simulink model "RichaLaika"  (R2025b)
settings: Solver=VariableStepAuto  StartTime=0.0  StopTime=10.0  RelTol=1e-3
undefined symbols (not defined in the file): ActivationSignal, ChargingWire, DataIN, DataOUT, OutputWire, SwitchSignal, TriggerSignal
settings Model: Creator=jakeo  LastModifiedBy=Richa

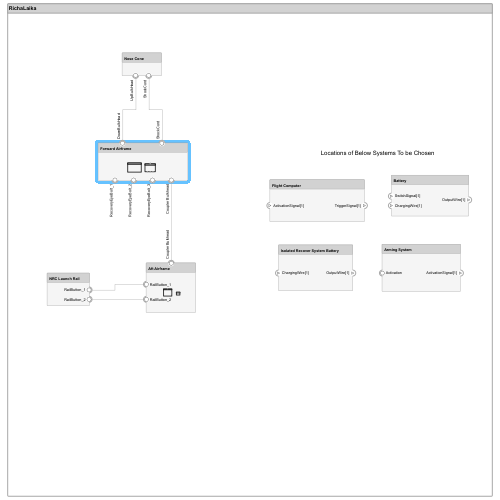
[thumbnail: Simulink's stored preview of the top-level diagram]
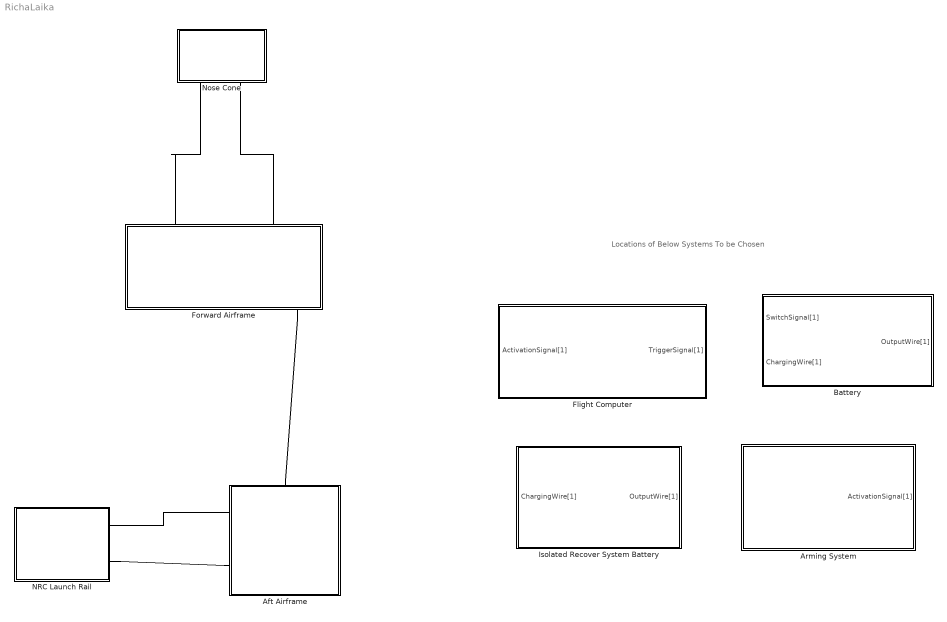
== system RichaLaika ==
  note: Locations of Below Systems To be Chosen
  Aft Airframe : Subsystem
      settings: PortSchema="{\"entries\":[{\"content\":{\"headerSize\":26,\"margin\":15,\"minimumSpacing\":25,\"sides\":[{\"content\":{\"connectorIds\":[\"LConn1\",\"LConn2\"]},\"type\":\"ConnectorPlacement.EquallySpacedRectSide\",\"uuid\":\"03e957df-4bae-46ab-9d0d-48f80a496ac5\"},{\"content\":{\"side\":\"RIGHT\"},\"type\":\"ConnectorPlacement.EquallySpacedRectSide\",\"uuid\":\"d2433d43-ba0e-4345-8a8e-99b57dcef125\"},{\"content\":{\"connectorIds\":[\"LConn3\"],\"side\":\"TOP\"},\"type\":\"ConnectorPlacement.EquallySpacedRectSide\",\"uuid\":\"84844adf-0e3d-439c-a28c-7cf27e8d243a\"},{\"content\":{\"side\":\"BOTTOM\"},\"type\":\"ConnectorPlacement.EquallySpacedRectSide\",\"uuid\":\"3d019cf0-7990-47c2-88c6-9af96c612354\"}]},\"type\":\"ConnectorPlacement.EquallySpacedConnector\",\"uuid\":\"9b26577b-50b2-4983-8f3c-4df87f23ba49\"}],\"packageUris\":[\"http://schema.mathworks.com/mf0/Connector/R2020b\"],\"version\":\"1.0\"}"
  Arming System : Subsystem
      settings: PortSchema="{\"entries\":[{\"content\":{\"headerSize\":26,\"margin\":15,\"minimumSpacing\":25,\"sides\":[{\"content\":{\"connectorIds\":[\"LConn1\"]},\"type\":\"ConnectorPlacement.EquallySpacedRectSide\",\"uuid\":\"6f4db608-f49c-4d1a-85cc-b66ec62c2f96\"},{\"content\":{\"connectorIds\":[\"Out1\"],\"side\":\"RIGHT\"},\"type\":\"ConnectorPlacement.EquallySpacedRectSide\",\"uuid\":\"3e275c67-1c5c-46cd-973f-75adcfca9e5d\"},{\"content\":{\"side\":\"TOP\"},\"type\":\"ConnectorPlacement.EquallySpacedRectSide\",\"uuid\":\"88fdcd36-c2bf-423f-a1bd-8e2b1c2ac438\"}]},\"type\":\"ConnectorPlacement.EquallySpacedConnector\",\"uuid\":\"596a3d77-8add-49e5-be48-e23e6a2b115a\"}],\"packageUris\":[\"http://schema.mathworks.com/mf0/Connector/R2020b\"],\"version\":\"1.0\"}"
  Battery : Subsystem
      settings: PortSchema="{\"entries\":[{\"content\":{\"headerSize\":26,\"margin\":15,\"minimumSpacing\":25,\"sides\":[{\"content\":{\"connectorIds\":[\"In1\",\"In2\"]},\"type\":\"ConnectorPlacement.EquallySpacedRectSide\",\"uuid\":\"03e957df-4bae-46ab-9d0d-48f80a496ac5\"},{\"content\":{\"connectorIds\":[\"Out1\"],\"side\":\"RIGHT\"},\"type\":\"ConnectorPlacement.EquallySpacedRectSide\",\"uuid\":\"d2433d43-ba0e-4345-8a8e-99b57dcef125\"},{\"content\":{\"side\":\"TOP\"},\"type\":\"ConnectorPlacement.EquallySpacedRectSide\",\"uuid\":\"84844adf-0e3d-439c-a28c-7cf27e8d243a\"}]},\"type\":\"ConnectorPlacement.EquallySpacedConnector\",\"uuid\":\"9b26577b-50b2-4983-8f3c-4df87f23ba49\"}],\"packageUris\":[\"http://schema.mathworks.com/mf0/Connector/R2020b\"],\"version\":\"1.0\"}"
  Flight Computer : Subsystem
      settings: PortSchema="{\"entries\":[{\"content\":{\"headerSize\":26,\"margin\":15,\"minimumSpacing\":25,\"sides\":[{\"content\":{\"connectorIds\":[\"In1\"]},\"type\":\"ConnectorPlacement.EquallySpacedRectSide\",\"uuid\":\"6f4db608-f49c-4d1a-85cc-b66ec62c2f96\"},{\"content\":{\"connectorIds\":[\"Out1\"],\"side\":\"RIGHT\"},\"type\":\"ConnectorPlacement.EquallySpacedRectSide\",\"uuid\":\"3e275c67-1c5c-46cd-973f-75adcfca9e5d\"},{\"content\":{\"side\":\"TOP\"},\"type\":\"ConnectorPlacement.EquallySpacedRectSide\",\"uuid\":\"88fdcd36-c2bf-423f-a1bd-8e2b1c2ac438\"}]},\"type\":\"ConnectorPlacement.EquallySpacedConnector\",\"uuid\":\"596a3d77-8add-49e5-be48-e23e6a2b115a\"}],\"packageUris\":[\"http://schema.mathworks.com/mf0/Connector/R2020b\"],\"version\":\"1.0\"}"
  Forward Airframe : Subsystem
      settings: PortSchema="{\"entries\":[{\"content\":{\"headerSize\":26,\"margin\":15,\"minimumSpacing\":25,\"sides\":[{\"content\":{},\"type\":\"ConnectorPlacement.EquallySpacedRectSide\",\"uuid\":\"03e957df-4bae-46ab-9d0d-48f80a496ac5\"},{\"content\":{\"side\":\"RIGHT\"},\"type\":\"ConnectorPlacement.EquallySpacedRectSide\",\"uuid\":\"d2433d43-ba0e-4345-8a8e-99b57dcef125\"},{\"content\":{\"connectorIds\":[\"LConn2\",\"LConn1\"],\"side\":\"TOP\"},\"type\":\"ConnectorPlacement.EquallySpacedRectSide\",\"uuid\":\"84844adf-0e3d-439c-a28c-7cf27e8d243a\"},{\"content\":{\"connectorIds\":[\"RConn2\",\"RConn3\",\"RConn4\",\"RConn1\"],\"side\":\"BOTTOM\"},\"type\":\"ConnectorPlacement.EquallySpacedRectSide\",\"uuid\":\"7d79bddd-aaf5-48a9-85da-385393746c36\"}]},\"type\":\"ConnectorPlacement.EquallySpacedConnector\",\"uuid\":\"9b26577b-50b2-4983-8f3c-4df87f23ba49\"}],\"packageUris\":[\"http://schema.mathworks.com/mf0/Connector/R2020b\"],\"version\":\"1.0\"}"
  Isolated Recover System Battery : Subsystem
      settings: PortSchema="{\"entries\":[{\"content\":{\"headerSize\":26,\"margin\":15,\"minimumSpacing\":25,\"sides\":[{\"content\":{\"connectorIds\":[\"In1\"]},\"type\":\"ConnectorPlacement.EquallySpacedRectSide\",\"uuid\":\"6f4db608-f49c-4d1a-85cc-b66ec62c2f96\"},{\"content\":{\"connectorIds\":[\"Out1\"],\"side\":\"RIGHT\"},\"type\":\"ConnectorPlacement.EquallySpacedRectSide\",\"uuid\":\"3e275c67-1c5c-46cd-973f-75adcfca9e5d\"},{\"content\":{\"side\":\"TOP\"},\"type\":\"ConnectorPlacement.EquallySpacedRectSide\",\"uuid\":\"88fdcd36-c2bf-423f-a1bd-8e2b1c2ac438\"}]},\"type\":\"ConnectorPlacement.EquallySpacedConnector\",\"uuid\":\"596a3d77-8add-49e5-be48-e23e6a2b115a\"}],\"packageUris\":[\"http://schema.mathworks.com/mf0/Connector/R2020b\"],\"version\":\"1.0\"}"
  NRC Launch Rail : Subsystem
      settings: PortSchema="{\"entries\":[{\"content\":{\"headerSize\":26,\"margin\":15,\"minimumSpacing\":25,\"sides\":[{\"content\":{},\"type\":\"ConnectorPlacement.EquallySpacedRectSide\",\"uuid\":\"6f4db608-f49c-4d1a-85cc-b66ec62c2f96\"},{\"content\":{\"connectorIds\":[\"RConn1\",\"RConn2\"],\"side\":\"RIGHT\"},\"type\":\"ConnectorPlacement.EquallySpacedRectSide\",\"uuid\":\"3e275c67-1c5c-46cd-973f-75adcfca9e5d\"},{\"content\":{\"side\":\"TOP\"},\"type\":\"ConnectorPlacement.EquallySpacedRectSide\",\"uuid\":\"88fdcd36-c2bf-423f-a1bd-8e2b1c2ac438\"}]},\"type\":\"ConnectorPlacement.EquallySpacedConnector\",\"uuid\":\"596a3d77-8add-49e5-be48-e23e6a2b115a\"}],\"packageUris\":[\"http://schema.mathworks.com/mf0/Connector/R2020b\"],\"version\":\"1.0\"}"
  Nose Cone : Subsystem
      settings: PortSchema="{\"entries\":[{\"content\":{\"headerSize\":26,\"margin\":15,\"minimumSpacing\":25,\"sides\":[{\"content\":{},\"type\":\"ConnectorPlacement.EquallySpacedRectSide\",\"uuid\":\"03e957df-4bae-46ab-9d0d-48f80a496ac5\"},{\"content\":{\"side\":\"RIGHT\"},\"type\":\"ConnectorPlacement.EquallySpacedRectSide\",\"uuid\":\"d2433d43-ba0e-4345-8a8e-99b57dcef125\"},{\"content\":{\"side\":\"TOP\"},\"type\":\"ConnectorPlacement.EquallySpacedRectSide\",\"uuid\":\"84844adf-0e3d-439c-a28c-7cf27e8d243a\"},{\"content\":{\"connectorIds\":[\"RConn1\",\"LConn1\"],\"side\":\"BOTTOM\"},\"type\":\"ConnectorPlacement.EquallySpacedRectSide\",\"uuid\":\"52e1799e-3f90-4e46-b959-6af2ed3cd00a\"}]},\"type\":\"ConnectorPlacement.EquallySpacedConnector\",\"uuid\":\"9b26577b-50b2-4983-8f3c-4df87f23ba49\"}],\"packageUris\":[\"http://schema.mathworks.com/mf0/Connector/R2020b\"],\"version\":\"1.0\"}"
  connections:
  Nose Cone/LConn1 -- Forward Airframe/LConn1
  Nose Cone/RConn1 -- Forward Airframe/LConn2
  NRC Launch Rail/RConn1 -- Aft Airframe/LConn1
  NRC Launch Rail/RConn2 -- Aft Airframe/LConn2
  Forward Airframe/RConn1 -- Aft Airframe/LConn3

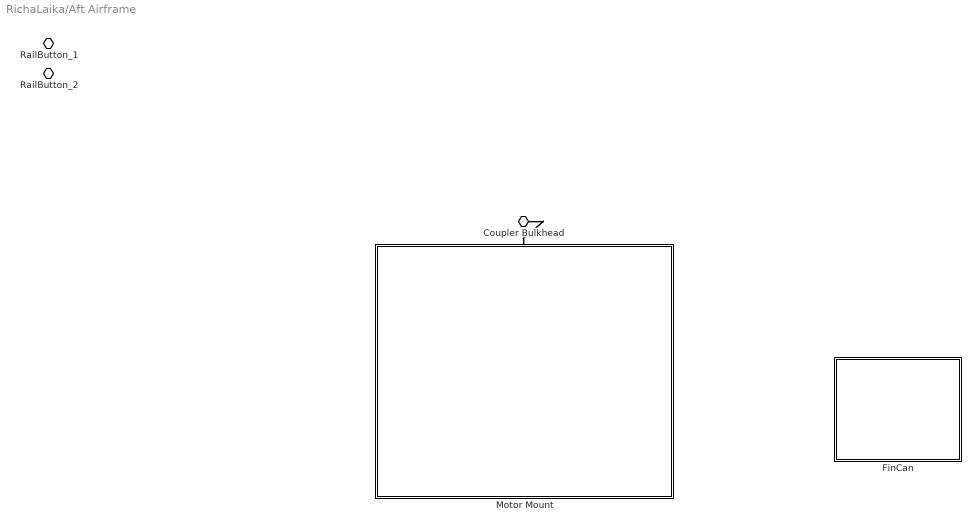
== system RichaLaika/Aft Airframe ==
  FinCan : Subsystem
      settings: PortSchema="{\"entries\":[{\"content\":{\"headerSize\":26,\"margin\":15,\"minimumSpacing\":25,\"sides\":[{\"content\":{},\"type\":\"ConnectorPlacement.EquallySpacedRectSide\",\"uuid\":\"b8130898-a228-4777-928b-c45fd71fae12\"},{\"content\":{\"side\":\"RIGHT\"},\"type\":\"ConnectorPlacement.EquallySpacedRectSide\",\"uuid\":\"2e534d82-eb77-4958-a6c7-3df50b0f76b8\"},{\"content\":{\"connectorIds\":[\"LConn1\",\"LConn2\",\"LConn3\",\"LConn4\"],\"side\":\"TOP\"},\"type\":\"ConnectorPlacement.EquallySpacedRectSide\",\"uuid\":\"3377e7dd-a415-4e95-88ef-4d0f5ef1cb04\"}]},\"type\":\"ConnectorPlacement.EquallySpacedConnector\",\"uuid\":\"f74309f9-da3e-4b22-b86a-0a2c471e6b03\"}],\"packageUris\":[\"http://schema.mathworks.com/mf0/Connector/R2020b\"],\"version\":\"1.0\"}"
  Motor Mount : Subsystem
      settings: PortSchema="{\"entries\":[{\"content\":{\"headerSize\":26,\"margin\":15,\"minimumSpacing\":25,\"sides\":[{\"content\":{},\"type\":\"ConnectorPlacement.EquallySpacedRectSide\",\"uuid\":\"31a1afce-5e8d-4ecd-8541-15d1c40c1f45\"},{\"content\":{\"connectorIds\":[\"LConn2\"],\"side\":\"RIGHT\"},\"type\":\"ConnectorPlacement.EquallySpacedRectSide\",\"uuid\":\"3ed7ed21-4334-432f-9367-bfee11c65601\"},{\"content\":{\"connectorIds\":[\"LConn1\"],\"side\":\"TOP\"},\"type\":\"ConnectorPlacement.EquallySpacedRectSide\",\"uuid\":\"099656eb-739b-474e-8ddd-dbd0ceba9a2b\"}]},\"type\":\"ConnectorPlacement.EquallySpacedConnector\",\"uuid\":\"a8320310-5044-4b61-8848-b99dff184188\"}],\"packageUris\":[\"http://schema.mathworks.com/mf0/Connector/R2020b\"],\"version\":\"1.0\"}"
  RailButton_1 : PMIOPort  Side=Left
  RailButton_2 : PMIOPort  Port=2  Side=Left
  Coupler Bulkhead : PMIOPort  Port=3  Side=Left
  connections:
  Coupler Bulkhead/RConn1 -- Motor Mount/LConn1

== system RichaLaika/Arming System ==
  Activation : PMIOPort  Side=Left
  Bus Element Out1 : Outport  PortName=ActivationSignal[1]

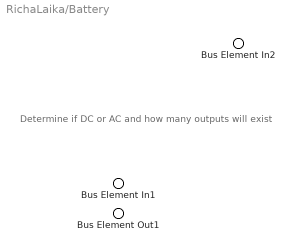
== system RichaLaika/Battery ==
  note: Determine if DC or AC and how many outputs will exist
  Bus Element In2 : Inport  PortName=SwitchSignal[1]
  Bus Element In1 : Inport  Port=2  PortName=ChargingWire[1]
  Bus Element Out1 : Outport  PortName=OutputWire[1]

== system RichaLaika/Flight Computer ==
  Bus Element In1 : Inport  PortName=ActivationSignal[1]
  Bus Element Out1 : Outport  PortName=TriggerSignal[1]

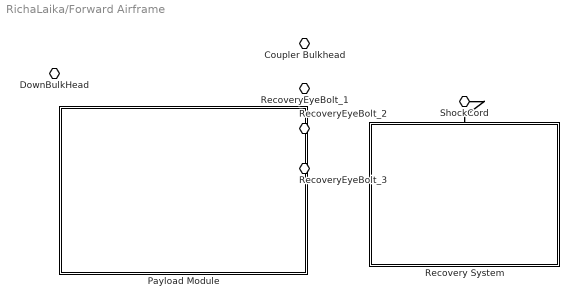
== system RichaLaika/Forward Airframe ==
  Payload Module : Subsystem
      settings: PortSchema="{\"entries\":[{\"content\":{\"headerSize\":26,\"margin\":15,\"minimumSpacing\":25,\"sides\":[{\"content\":{},\"type\":\"ConnectorPlacement.EquallySpacedRectSide\",\"uuid\":\"31a1afce-5e8d-4ecd-8541-15d1c40c1f45\"},{\"content\":{\"side\":\"RIGHT\"},\"type\":\"ConnectorPlacement.EquallySpacedRectSide\",\"uuid\":\"3ed7ed21-4334-432f-9367-bfee11c65601\"},{\"content\":{\"side\":\"TOP\"},\"type\":\"ConnectorPlacement.EquallySpacedRectSide\",\"uuid\":\"099656eb-739b-474e-8ddd-dbd0ceba9a2b\"}]},\"type\":\"ConnectorPlacement.EquallySpacedConnector\",\"uuid\":\"a8320310-5044-4b61-8848-b99dff184188\"}],\"packageUris\":[\"http://schema.mathworks.com/mf0/Connector/R2020b\"],\"version\":\"1.0\"}"
  Recovery System : Subsystem
      settings: PortSchema="{\"entries\":[{\"content\":{\"headerSize\":26,\"margin\":15,\"minimumSpacing\":25,\"sides\":[{\"content\":{},\"type\":\"ConnectorPlacement.EquallySpacedRectSide\",\"uuid\":\"31a1afce-5e8d-4ecd-8541-15d1c40c1f45\"},{\"content\":{\"side\":\"RIGHT\"},\"type\":\"ConnectorPlacement.EquallySpacedRectSide\",\"uuid\":\"3ed7ed21-4334-432f-9367-bfee11c65601\"},{\"content\":{\"connectorIds\":[\"LConn1\"],\"side\":\"TOP\"},\"type\":\"ConnectorPlacement.EquallySpacedRectSide\",\"uuid\":\"099656eb-739b-474e-8ddd-dbd0ceba9a2b\"},{\"content\":{\"connectorIds\":[\"RConn3\",\"RConn1\",\"RConn2\"],\"side\":\"BOTTOM\"},\"type\":\"ConnectorPlacement.EquallySpacedRectSide\",\"uuid\":\"aa9f3616-ef86-4a01-82fa-8dfdf1ff0ef2\"}]},\"type\":\"ConnectorPlacement.EquallySpacedConnector\",\"uuid\":\"a8320310-5044-4b61-8848-b99dff184188\"}],\"packageUris\":[\"http://schema.mathworks.com/mf0/Connector/R2020b\"],\"version\":\"1.0\"}"
  ShockCord : PMIOPort  Side=Left
  DownBulkHead : PMIOPort  Port=2  Side=Left
  Coupler Bulkhead : PMIOPort  Port=3  Side=Right
  RecoveryEyeBolt_1 : PMIOPort  Port=4  Side=Right
  RecoveryEyeBolt_2 : PMIOPort  Port=5  Side=Right
  RecoveryEyeBolt_3 : PMIOPort  Port=6  Side=Right
  connections:
  ShockCord/RConn1 -- Recovery System/LConn1

== system RichaLaika/Isolated Recover System Battery ==
  Bus Element In1 : Inport  PortName=ChargingWire[1]
  Bus Element Out1 : Outport  PortName=OutputWire[1]

== system RichaLaika/NRC Launch Rail ==
  RailButton_1 : PMIOPort  Side=Right
  RailButton_2 : PMIOPort  Port=2  Side=Right

== system RichaLaika/Nose Cone ==
  ShockCord : PMIOPort  Side=Left
  UpBulkHead : PMIOPort  Port=2  Side=Right

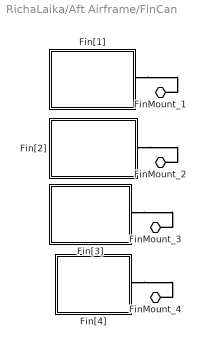
== system RichaLaika/Aft Airframe/FinCan ==
  Fin[1] : Subsystem
      settings: PortSchema="{\"entries\":[{\"content\":{\"headerSize\":26,\"margin\":15,\"minimumSpacing\":25,\"sides\":[{\"content\":{},\"type\":\"ConnectorPlacement.EquallySpacedRectSide\",\"uuid\":\"03e957df-4bae-46ab-9d0d-48f80a496ac5\"},{\"content\":{\"connectorIds\":[\"LConn1\"],\"side\":\"RIGHT\"},\"type\":\"ConnectorPlacement.EquallySpacedRectSide\",\"uuid\":\"d2433d43-ba0e-4345-8a8e-99b57dcef125\"},{\"content\":{\"side\":\"TOP\"},\"type\":\"ConnectorPlacement.EquallySpacedRectSide\",\"uuid\":\"84844adf-0e3d-439c-a28c-7cf27e8d243a\"}]},\"type\":\"ConnectorPlacement.EquallySpacedConnector\",\"uuid\":\"9b26577b-50b2-4983-8f3c-4df87f23ba49\"}],\"packageUris\":[\"http://schema.mathworks.com/mf0/Connector/R2020b\"],\"version\":\"1.0\"}"
  Fin[2] : Subsystem
      settings: PortSchema="{\"entries\":[{\"content\":{\"headerSize\":26,\"margin\":15,\"minimumSpacing\":25,\"sides\":[{\"content\":{},\"type\":\"ConnectorPlacement.EquallySpacedRectSide\",\"uuid\":\"03e957df-4bae-46ab-9d0d-48f80a496ac5\"},{\"content\":{\"connectorIds\":[\"LConn1\"],\"side\":\"RIGHT\"},\"type\":\"ConnectorPlacement.EquallySpacedRectSide\",\"uuid\":\"d2433d43-ba0e-4345-8a8e-99b57dcef125\"},{\"content\":{\"side\":\"TOP\"},\"type\":\"ConnectorPlacement.EquallySpacedRectSide\",\"uuid\":\"84844adf-0e3d-439c-a28c-7cf27e8d243a\"}]},\"type\":\"ConnectorPlacement.EquallySpacedConnector\",\"uuid\":\"9b26577b-50b2-4983-8f3c-4df87f23ba49\"}],\"packageUris\":[\"http://schema.mathworks.com/mf0/Connector/R2020b\"],\"version\":\"1.0\"}"
  Fin[3] : Subsystem
      settings: PortSchema="{\"entries\":[{\"content\":{\"headerSize\":26,\"margin\":15,\"minimumSpacing\":25,\"sides\":[{\"content\":{},\"type\":\"ConnectorPlacement.EquallySpacedRectSide\",\"uuid\":\"03e957df-4bae-46ab-9d0d-48f80a496ac5\"},{\"content\":{\"connectorIds\":[\"LConn1\"],\"side\":\"RIGHT\"},\"type\":\"ConnectorPlacement.EquallySpacedRectSide\",\"uuid\":\"d2433d43-ba0e-4345-8a8e-99b57dcef125\"},{\"content\":{\"side\":\"TOP\"},\"type\":\"ConnectorPlacement.EquallySpacedRectSide\",\"uuid\":\"84844adf-0e3d-439c-a28c-7cf27e8d243a\"}]},\"type\":\"ConnectorPlacement.EquallySpacedConnector\",\"uuid\":\"9b26577b-50b2-4983-8f3c-4df87f23ba49\"}],\"packageUris\":[\"http://schema.mathworks.com/mf0/Connector/R2020b\"],\"version\":\"1.0\"}"
  Fin[4] : Subsystem
      settings: PortSchema="{\"entries\":[{\"content\":{\"headerSize\":26,\"margin\":15,\"minimumSpacing\":25,\"sides\":[{\"content\":{},\"type\":\"ConnectorPlacement.EquallySpacedRectSide\",\"uuid\":\"03e957df-4bae-46ab-9d0d-48f80a496ac5\"},{\"content\":{\"connectorIds\":[\"LConn1\"],\"side\":\"RIGHT\"},\"type\":\"ConnectorPlacement.EquallySpacedRectSide\",\"uuid\":\"d2433d43-ba0e-4345-8a8e-99b57dcef125\"},{\"content\":{\"side\":\"TOP\"},\"type\":\"ConnectorPlacement.EquallySpacedRectSide\",\"uuid\":\"84844adf-0e3d-439c-a28c-7cf27e8d243a\"}]},\"type\":\"ConnectorPlacement.EquallySpacedConnector\",\"uuid\":\"9b26577b-50b2-4983-8f3c-4df87f23ba49\"}],\"packageUris\":[\"http://schema.mathworks.com/mf0/Connector/R2020b\"],\"version\":\"1.0\"}"
  FinMount_1 : PMIOPort  Side=Left
  FinMount_2 : PMIOPort  Port=2  Side=Left
  FinMount_3 : PMIOPort  Port=3  Side=Left
  FinMount_4 : PMIOPort  Port=4  Side=Left
  connections:
  Fin[1]/LConn1 -- FinMount_1/RConn1
  Fin[2]/LConn1 -- FinMount_2/RConn1
  Fin[3]/LConn1 -- FinMount_3/RConn1
  Fin[4]/LConn1 -- FinMount_4/RConn1

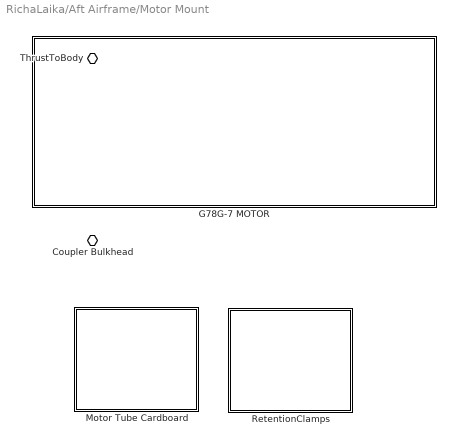
== system RichaLaika/Aft Airframe/Motor Mount ==
  G78G-7 MOTOR : Subsystem
      settings: PortSchema="{\"entries\":[{\"content\":{\"headerSize\":26,\"margin\":15,\"minimumSpacing\":25,\"sides\":[{\"content\":{\"connectorIds\":[\"LConn1\",\"LConn2\"]},\"type\":\"ConnectorPlacement.EquallySpacedRectSide\",\"uuid\":\"03e957df-4bae-46ab-9d0d-48f80a496ac5\"},{\"content\":{\"side\":\"RIGHT\"},\"type\":\"ConnectorPlacement.EquallySpacedRectSide\",\"uuid\":\"d2433d43-ba0e-4345-8a8e-99b57dcef125\"},{\"content\":{\"side\":\"TOP\"},\"type\":\"ConnectorPlacement.EquallySpacedRectSide\",\"uuid\":\"84844adf-0e3d-439c-a28c-7cf27e8d243a\"}]},\"type\":\"ConnectorPlacement.EquallySpacedConnector\",\"uuid\":\"9b26577b-50b2-4983-8f3c-4df87f23ba49\"}],\"packageUris\":[\"http://schema.mathworks.com/mf0/Connector/R2020b\"],\"version\":\"1.0\"}"
  Motor Tube Cardboard : Subsystem
      settings: PortSchema="{\"entries\":[{\"content\":{\"headerSize\":26,\"margin\":15,\"minimumSpacing\":25,\"sides\":[{\"content\":{},\"type\":\"ConnectorPlacement.EquallySpacedRectSide\",\"uuid\":\"b8130898-a228-4777-928b-c45fd71fae12\"},{\"content\":{\"side\":\"RIGHT\"},\"type\":\"ConnectorPlacement.EquallySpacedRectSide\",\"uuid\":\"2e534d82-eb77-4958-a6c7-3df50b0f76b8\"},{\"content\":{\"side\":\"TOP\"},\"type\":\"ConnectorPlacement.EquallySpacedRectSide\",\"uuid\":\"3377e7dd-a415-4e95-88ef-4d0f5ef1cb04\"}]},\"type\":\"ConnectorPlacement.EquallySpacedConnector\",\"uuid\":\"f74309f9-da3e-4b22-b86a-0a2c471e6b03\"}],\"packageUris\":[\"http://schema.mathworks.com/mf0/Connector/R2020b\"],\"version\":\"1.0\"}"
  RetentionClamps : Subsystem
      settings: PortSchema="{\"entries\":[{\"content\":{\"headerSize\":26,\"margin\":15,\"minimumSpacing\":25,\"sides\":[{\"content\":{},\"type\":\"ConnectorPlacement.EquallySpacedRectSide\",\"uuid\":\"b8130898-a228-4777-928b-c45fd71fae12\"},{\"content\":{\"side\":\"RIGHT\"},\"type\":\"ConnectorPlacement.EquallySpacedRectSide\",\"uuid\":\"2e534d82-eb77-4958-a6c7-3df50b0f76b8\"},{\"content\":{\"side\":\"TOP\"},\"type\":\"ConnectorPlacement.EquallySpacedRectSide\",\"uuid\":\"3377e7dd-a415-4e95-88ef-4d0f5ef1cb04\"}]},\"type\":\"ConnectorPlacement.EquallySpacedConnector\",\"uuid\":\"f74309f9-da3e-4b22-b86a-0a2c471e6b03\"}],\"packageUris\":[\"http://schema.mathworks.com/mf0/Connector/R2020b\"],\"version\":\"1.0\"}"
  Coupler Bulkhead : PMIOPort  Side=Left
  ThrustToBody : PMIOPort  Port=2  Side=Left

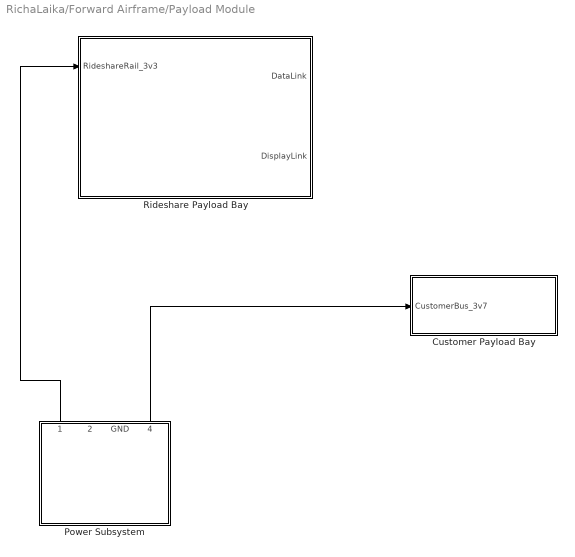
== system RichaLaika/Forward Airframe/Payload Module ==
  Customer Payload Bay : Subsystem
      settings: PortSchema="{\"entries\":[{\"content\":{\"headerSize\":26,\"margin\":15,\"minimumSpacing\":25,\"sides\":[{\"content\":{\"connectorIds\":[\"In1\"]},\"type\":\"ConnectorPlacement.EquallySpacedRectSide\",\"uuid\":\"03e957df-4bae-46ab-9d0d-48f80a496ac5\"},{\"content\":{\"side\":\"RIGHT\"},\"type\":\"ConnectorPlacement.EquallySpacedRectSide\",\"uuid\":\"d2433d43-ba0e-4345-8a8e-99b57dcef125\"},{\"content\":{\"side\":\"TOP\"},\"type\":\"ConnectorPlacement.EquallySpacedRectSide\",\"uuid\":\"84844adf-0e3d-439c-a28c-7cf27e8d243a\"}]},\"type\":\"ConnectorPlacement.EquallySpacedConnector\",\"uuid\":\"9b26577b-50b2-4983-8f3c-4df87f23ba49\"}],\"packageUris\":[\"http://schema.mathworks.com/mf0/Connector/R2020b\"],\"version\":\"1.0\"}"
  Power Subsystem : Subsystem
      settings: PortSchema="{\"entries\":[{\"content\":{\"headerSize\":26,\"margin\":15,\"minimumSpacing\":25,\"sides\":[{\"content\":{},\"type\":\"ConnectorPlacement.EquallySpacedRectSide\",\"uuid\":\"31a1afce-5e8d-4ecd-8541-15d1c40c1f45\"},{\"content\":{\"side\":\"RIGHT\"},\"type\":\"ConnectorPlacement.EquallySpacedRectSide\",\"uuid\":\"3ed7ed21-4334-432f-9367-bfee11c65601\"},{\"content\":{\"connectorIds\":[\"Out1\",\"Out2\",\"Out3\",\"Out4\"],\"side\":\"TOP\"},\"type\":\"ConnectorPlacement.EquallySpacedRectSide\",\"uuid\":\"099656eb-739b-474e-8ddd-dbd0ceba9a2b\"}]},\"type\":\"ConnectorPlacement.EquallySpacedConnector\",\"uuid\":\"a8320310-5044-4b61-8848-b99dff184188\"}],\"packageUris\":[\"http://schema.mathworks.com/mf0/Connector/R2020b\"],\"version\":\"1.0\"}"
  Rideshare Payload Bay : Subsystem
      settings: PortSchema="{\"entries\":[{\"content\":{\"headerSize\":26,\"margin\":15,\"minimumSpacing\":25,\"sides\":[{\"content\":{\"connectorIds\":[\"In1\",\"LConn1\",\"LConn2\"]},\"type\":\"ConnectorPlacement.EquallySpacedRectSide\",\"uuid\":\"03e957df-4bae-46ab-9d0d-48f80a496ac5\"},{\"content\":{\"connectorIds\":[\"Out1\",\"Out2\"],\"side\":\"RIGHT\"},\"type\":\"ConnectorPlacement.EquallySpacedRectSide\",\"uuid\":\"d2433d43-ba0e-4345-8a8e-99b57dcef125\"},{\"content\":{\"side\":\"TOP\"},\"type\":\"ConnectorPlacement.EquallySpacedRectSide\",\"uuid\":\"84844adf-0e3d-439c-a28c-7cf27e8d243a\"}]},\"type\":\"ConnectorPlacement.EquallySpacedConnector\",\"uuid\":\"9b26577b-50b2-4983-8f3c-4df87f23ba49\"}],\"packageUris\":[\"http://schema.mathworks.com/mf0/Connector/R2020b\"],\"version\":\"1.0\"}"
  wires:
  Power Subsystem/1(RideshareRail_3v3) -> Rideshare Payload Bay/1(RideshareRail_3v3)
  Power Subsystem/4(CustomerBus_3v7) -> Customer Payload Bay/1(CustomerBus_3v7)

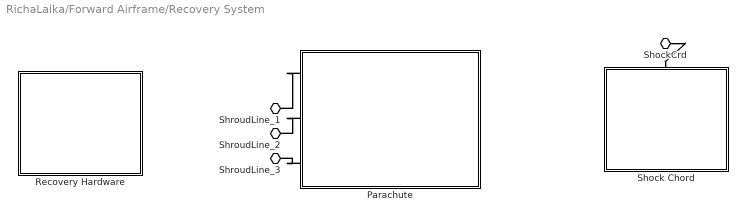
== system RichaLaika/Forward Airframe/Recovery System ==
  Parachute : Subsystem
      settings: PortSchema="{\"entries\":[{\"content\":{\"headerSize\":26,\"margin\":15,\"minimumSpacing\":25,\"sides\":[{\"content\":{\"connectorIds\":[\"LConn1\",\"LConn2\",\"LConn3\"]},\"type\":\"ConnectorPlacement.EquallySpacedRectSide\",\"uuid\":\"03e957df-4bae-46ab-9d0d-48f80a496ac5\"},{\"content\":{\"side\":\"RIGHT\"},\"type\":\"ConnectorPlacement.EquallySpacedRectSide\",\"uuid\":\"d2433d43-ba0e-4345-8a8e-99b57dcef125\"},{\"content\":{\"side\":\"TOP\"},\"type\":\"ConnectorPlacement.EquallySpacedRectSide\",\"uuid\":\"84844adf-0e3d-439c-a28c-7cf27e8d243a\"}]},\"type\":\"ConnectorPlacement.EquallySpacedConnector\",\"uuid\":\"9b26577b-50b2-4983-8f3c-4df87f23ba49\"}],\"packageUris\":[\"http://schema.mathworks.com/mf0/Connector/R2020b\"],\"version\":\"1.0\"}"
  Recovery Hardware : Subsystem
      settings: PortSchema="{\"entries\":[{\"content\":{\"headerSize\":26,\"margin\":15,\"minimumSpacing\":25,\"sides\":[{\"content\":{},\"type\":\"ConnectorPlacement.EquallySpacedRectSide\",\"uuid\":\"31a1afce-5e8d-4ecd-8541-15d1c40c1f45\"},{\"content\":{\"side\":\"RIGHT\"},\"type\":\"ConnectorPlacement.EquallySpacedRectSide\",\"uuid\":\"3ed7ed21-4334-432f-9367-bfee11c65601\"},{\"content\":{\"side\":\"TOP\"},\"type\":\"ConnectorPlacement.EquallySpacedRectSide\",\"uuid\":\"099656eb-739b-474e-8ddd-dbd0ceba9a2b\"}]},\"type\":\"ConnectorPlacement.EquallySpacedConnector\",\"uuid\":\"a8320310-5044-4b61-8848-b99dff184188\"}],\"packageUris\":[\"http://schema.mathworks.com/mf0/Connector/R2020b\"],\"version\":\"1.0\"}"
  Shock Chord : Subsystem
      settings: PortSchema="{\"entries\":[{\"content\":{\"headerSize\":26,\"margin\":15,\"minimumSpacing\":25,\"sides\":[{\"content\":{},\"type\":\"ConnectorPlacement.EquallySpacedRectSide\",\"uuid\":\"31a1afce-5e8d-4ecd-8541-15d1c40c1f45\"},{\"content\":{\"side\":\"RIGHT\"},\"type\":\"ConnectorPlacement.EquallySpacedRectSide\",\"uuid\":\"3ed7ed21-4334-432f-9367-bfee11c65601\"},{\"content\":{\"connectorIds\":[\"LConn1\"],\"side\":\"TOP\"},\"type\":\"ConnectorPlacement.EquallySpacedRectSide\",\"uuid\":\"099656eb-739b-474e-8ddd-dbd0ceba9a2b\"}]},\"type\":\"ConnectorPlacement.EquallySpacedConnector\",\"uuid\":\"a8320310-5044-4b61-8848-b99dff184188\"}],\"packageUris\":[\"http://schema.mathworks.com/mf0/Connector/R2020b\"],\"version\":\"1.0\"}"
  ShockCrd : PMIOPort  Side=Left
  ShroudLine_2 : PMIOPort  Port=2  Side=Right
  ShroudLine_3 : PMIOPort  Port=3  Side=Right
  ShroudLine_1 : PMIOPort  Port=4  Side=Right
  connections:
  ShockCrd/RConn1 -- Shock Chord/LConn1
  Parachute/LConn1 -- ShroudLine_1/RConn1
  Parachute/LConn2 -- ShroudLine_2/RConn1
  Parachute/LConn3 -- ShroudLine_3/RConn1

== system RichaLaika/Aft Airframe/FinCan/Fin[1] ==
  FinMount[1] : PMIOPort  Side=Left

== system RichaLaika/Aft Airframe/FinCan/Fin[2] ==
  FinMount[2] : PMIOPort  Side=Left

== system RichaLaika/Aft Airframe/FinCan/Fin[3] ==
  FinMount[3] : PMIOPort  Side=Left

== system RichaLaika/Aft Airframe/FinCan/Fin[4] ==
  FinMount[4] : PMIOPort  Side=Left

== system RichaLaika/Aft Airframe/Motor Mount/G78G-7 MOTOR ==
  Mount[1] : PMIOPort  Side=Left
  Mount[2] : PMIOPort  Port=2  Side=Left

== system RichaLaika/Aft Airframe/Motor Mount/Motor Tube Cardboard ==

== system RichaLaika/Aft Airframe/Motor Mount/RetentionClamps ==

== system RichaLaika/Forward Airframe/Payload Module/Customer Payload Bay ==
  Bus Element In2 : Inport  PortName=CustomerBus_3v7
  Customer Payload : Subsystem
      settings: PortSchema="{\"entries\":[{\"content\":{\"headerSize\":26,\"margin\":15,\"minimumSpacing\":25,\"sides\":[{\"content\":{\"connectorIds\":[\"In1\"]},\"type\":\"ConnectorPlacement.EquallySpacedRectSide\",\"uuid\":\"03e957df-4bae-46ab-9d0d-48f80a496ac5\"},{\"content\":{\"side\":\"RIGHT\"},\"type\":\"ConnectorPlacement.EquallySpacedRectSide\",\"uuid\":\"d2433d43-ba0e-4345-8a8e-99b57dcef125\"},{\"content\":{\"side\":\"TOP\"},\"type\":\"ConnectorPlacement.EquallySpacedRectSide\",\"uuid\":\"84844adf-0e3d-439c-a28c-7cf27e8d243a\"}]},\"type\":\"ConnectorPlacement.EquallySpacedConnector\",\"uuid\":\"9b26577b-50b2-4983-8f3c-4df87f23ba49\"}],\"packageUris\":[\"http://schema.mathworks.com/mf0/Connector/R2020b\"],\"version\":\"1.0\"}"
  Male XT30 Connector : Subsystem
      settings: PortSchema="{\"entries\":[{\"content\":{\"headerSize\":26,\"margin\":15,\"minimumSpacing\":25,\"sides\":[{\"content\":{\"connectorIds\":[\"In1\"]},\"type\":\"ConnectorPlacement.EquallySpacedRectSide\",\"uuid\":\"31a1afce-5e8d-4ecd-8541-15d1c40c1f45\"},{\"content\":{\"connectorIds\":[\"Out1\"],\"side\":\"RIGHT\"},\"type\":\"ConnectorPlacement.EquallySpacedRectSide\",\"uuid\":\"3ed7ed21-4334-432f-9367-bfee11c65601\"},{\"content\":{\"side\":\"TOP\"},\"type\":\"ConnectorPlacement.EquallySpacedRectSide\",\"uuid\":\"099656eb-739b-474e-8ddd-dbd0ceba9a2b\"}]},\"type\":\"ConnectorPlacement.EquallySpacedConnector\",\"uuid\":\"a8320310-5044-4b61-8848-b99dff184188\"}],\"packageUris\":[\"http://schema.mathworks.com/mf0/Connector/R2020b\"],\"version\":\"1.0\"}"
  wires:
  Male XT30 Connector/1(Customer Payload Connector) -> Customer Payload/1(Customer Payload Connector)
  Bus Element In2/1 -> Male XT30 Connector/1(CustomerBus_3v7)

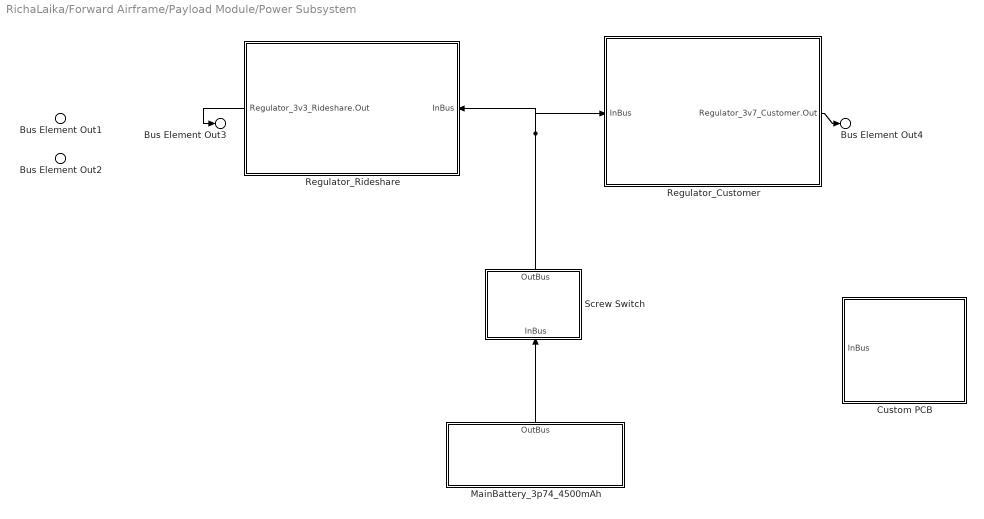
== system RichaLaika/Forward Airframe/Payload Module/Power Subsystem ==
  Custom PCB : Subsystem
      settings: PortSchema="{\"entries\":[{\"content\":{\"headerSize\":26,\"margin\":15,\"minimumSpacing\":25,\"sides\":[{\"content\":{\"connectorIds\":[\"In1\"]},\"type\":\"ConnectorPlacement.EquallySpacedRectSide\",\"uuid\":\"31a1afce-5e8d-4ecd-8541-15d1c40c1f45\"},{\"content\":{\"side\":\"RIGHT\"},\"type\":\"ConnectorPlacement.EquallySpacedRectSide\",\"uuid\":\"3ed7ed21-4334-432f-9367-bfee11c65601\"},{\"content\":{\"side\":\"TOP\"},\"type\":\"ConnectorPlacement.EquallySpacedRectSide\",\"uuid\":\"099656eb-739b-474e-8ddd-dbd0ceba9a2b\"}]},\"type\":\"ConnectorPlacement.EquallySpacedConnector\",\"uuid\":\"a8320310-5044-4b61-8848-b99dff184188\"}],\"packageUris\":[\"http://schema.mathworks.com/mf0/Connector/R2020b\"],\"version\":\"1.0\"}"
  MainBattery_3p74_4500mAh : Subsystem
      settings: PortSchema="{\"entries\":[{\"content\":{\"headerSize\":26,\"margin\":15,\"minimumSpacing\":25,\"sides\":[{\"content\":{},\"type\":\"ConnectorPlacement.EquallySpacedRectSide\",\"uuid\":\"31a1afce-5e8d-4ecd-8541-15d1c40c1f45\"},{\"content\":{\"side\":\"RIGHT\"},\"type\":\"ConnectorPlacement.EquallySpacedRectSide\",\"uuid\":\"3ed7ed21-4334-432f-9367-bfee11c65601\"},{\"content\":{\"connectorIds\":[\"Out1\"],\"side\":\"TOP\"},\"type\":\"ConnectorPlacement.EquallySpacedRectSide\",\"uuid\":\"099656eb-739b-474e-8ddd-dbd0ceba9a2b\"}]},\"type\":\"ConnectorPlacement.EquallySpacedConnector\",\"uuid\":\"a8320310-5044-4b61-8848-b99dff184188\"}],\"packageUris\":[\"http://schema.mathworks.com/mf0/Connector/R2020b\"],\"version\":\"1.0\"}"
  Regulator_Customer : Subsystem
      settings: PortSchema="{\"entries\":[{\"content\":{\"headerSize\":26,\"margin\":15,\"minimumSpacing\":25,\"sides\":[{\"content\":{\"connectorIds\":[\"In1\"]},\"type\":\"ConnectorPlacement.EquallySpacedRectSide\",\"uuid\":\"31a1afce-5e8d-4ecd-8541-15d1c40c1f45\"},{\"content\":{\"connectorIds\":[\"Out1\"],\"side\":\"RIGHT\"},\"type\":\"ConnectorPlacement.EquallySpacedRectSide\",\"uuid\":\"3ed7ed21-4334-432f-9367-bfee11c65601\"},{\"content\":{\"side\":\"TOP\"},\"type\":\"ConnectorPlacement.EquallySpacedRectSide\",\"uuid\":\"099656eb-739b-474e-8ddd-dbd0ceba9a2b\"}]},\"type\":\"ConnectorPlacement.EquallySpacedConnector\",\"uuid\":\"a8320310-5044-4b61-8848-b99dff184188\"}],\"packageUris\":[\"http://schema.mathworks.com/mf0/Connector/R2020b\"],\"version\":\"1.0\"}"
  Regulator_Rideshare : Subsystem
      settings: PortSchema="{\"entries\":[{\"content\":{\"headerSize\":26,\"margin\":15,\"minimumSpacing\":25,\"sides\":[{\"content\":{\"connectorIds\":[\"Out1\"]},\"type\":\"ConnectorPlacement.EquallySpacedRectSide\",\"uuid\":\"31a1afce-5e8d-4ecd-8541-15d1c40c1f45\"},{\"content\":{\"connectorIds\":[\"In1\"],\"side\":\"RIGHT\"},\"type\":\"ConnectorPlacement.EquallySpacedRectSide\",\"uuid\":\"3ed7ed21-4334-432f-9367-bfee11c65601\"},{\"content\":{\"side\":\"TOP\"},\"type\":\"ConnectorPlacement.EquallySpacedRectSide\",\"uuid\":\"099656eb-739b-474e-8ddd-dbd0ceba9a2b\"}]},\"type\":\"ConnectorPlacement.EquallySpacedConnector\",\"uuid\":\"a8320310-5044-4b61-8848-b99dff184188\"}],\"packageUris\":[\"http://schema.mathworks.com/mf0/Connector/R2020b\"],\"version\":\"1.0\"}"
  Screw Switch : Subsystem
      settings: PortSchema="{\"entries\":[{\"content\":{\"headerSize\":26,\"margin\":15,\"minimumSpacing\":25,\"sides\":[{\"content\":{},\"type\":\"ConnectorPlacement.EquallySpacedRectSide\",\"uuid\":\"31a1afce-5e8d-4ecd-8541-15d1c40c1f45\"},{\"content\":{\"side\":\"RIGHT\"},\"type\":\"ConnectorPlacement.EquallySpacedRectSide\",\"uuid\":\"3ed7ed21-4334-432f-9367-bfee11c65601\"},{\"content\":{\"connectorIds\":[\"Out1\"],\"side\":\"TOP\"},\"type\":\"ConnectorPlacement.EquallySpacedRectSide\",\"uuid\":\"099656eb-739b-474e-8ddd-dbd0ceba9a2b\"},{\"content\":{\"connectorIds\":[\"In1\"],\"side\":\"BOTTOM\"},\"type\":\"ConnectorPlacement.EquallySpacedRectSide\",\"uuid\":\"624bbe72-623d-4402-8d5f-f41297524299\"}]},\"type\":\"ConnectorPlacement.EquallySpacedConnector\",\"uuid\":\"a8320310-5044-4b61-8848-b99dff184188\"}],\"packageUris\":[\"http://schema.mathworks.com/mf0/Connector/R2020b\"],\"version\":\"1.0\"}"
  Bus Element Out3 : Outport  PortName=RideshareRail_3v3
  Bus Element Out1 : Outport  Port=2  PortName=BatteryOut
  Bus Element Out2 : Outport  Port=3  PortName=GND
  Bus Element Out4 : Outport  Port=4  PortName=CustomerBus_3v7
  wires:
  MainBattery_3p74_4500mAh/1(OutBus) -> Screw Switch/1(InBus)
  Screw Switch/1(OutBus) -> Regulator_Customer/1(InBus), Regulator_Rideshare/1(InBus)
  Regulator_Rideshare/1(Regulator_3v3_Rideshare.Out) -> Bus Element Out3/1
  Regulator_Customer/1(Regulator_3v7_Customer.Out) -> Bus Element Out4/1

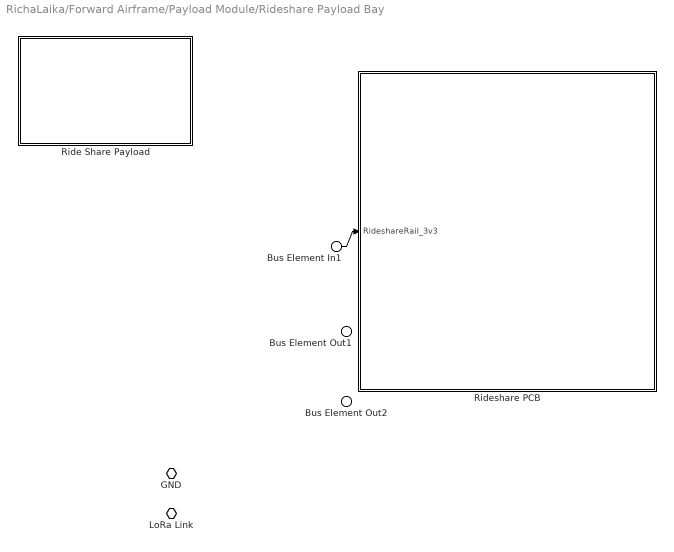
== system RichaLaika/Forward Airframe/Payload Module/Rideshare Payload Bay ==
  Bus Element In1 : Inport  PortName=RideshareRail_3v3
  Ride Share Payload : Subsystem
      settings: PortSchema="{\"entries\":[{\"content\":{\"headerSize\":26,\"margin\":15,\"minimumSpacing\":25,\"sides\":[{\"content\":{},\"type\":\"ConnectorPlacement.EquallySpacedRectSide\",\"uuid\":\"03e957df-4bae-46ab-9d0d-48f80a496ac5\"},{\"content\":{\"side\":\"RIGHT\"},\"type\":\"ConnectorPlacement.EquallySpacedRectSide\",\"uuid\":\"d2433d43-ba0e-4345-8a8e-99b57dcef125\"},{\"content\":{\"side\":\"TOP\"},\"type\":\"ConnectorPlacement.EquallySpacedRectSide\",\"uuid\":\"84844adf-0e3d-439c-a28c-7cf27e8d243a\"}]},\"type\":\"ConnectorPlacement.EquallySpacedConnector\",\"uuid\":\"9b26577b-50b2-4983-8f3c-4df87f23ba49\"}],\"packageUris\":[\"http://schema.mathworks.com/mf0/Connector/R2020b\"],\"version\":\"1.0\"}"
  Rideshare PCB : Subsystem
      settings: PortSchema="{\"entries\":[{\"content\":{\"headerSize\":26,\"margin\":15,\"minimumSpacing\":25,\"sides\":[{\"content\":{\"connectorIds\":[\"In1\"]},\"type\":\"ConnectorPlacement.EquallySpacedRectSide\",\"uuid\":\"b8130898-a228-4777-928b-c45fd71fae12\"},{\"content\":{\"side\":\"RIGHT\"},\"type\":\"ConnectorPlacement.EquallySpacedRectSide\",\"uuid\":\"2e534d82-eb77-4958-a6c7-3df50b0f76b8\"},{\"content\":{\"side\":\"TOP\"},\"type\":\"ConnectorPlacement.EquallySpacedRectSide\",\"uuid\":\"3377e7dd-a415-4e95-88ef-4d0f5ef1cb04\"}]},\"type\":\"ConnectorPlacement.EquallySpacedConnector\",\"uuid\":\"f74309f9-da3e-4b22-b86a-0a2c471e6b03\"}],\"packageUris\":[\"http://schema.mathworks.com/mf0/Connector/R2020b\"],\"version\":\"1.0\"}"
  GND : PMIOPort  Side=Left
  LoRa Link : PMIOPort  Port=2  Side=Left
  Bus Element Out1 : Outport  PortName=DataLink
  Bus Element Out2 : Outport  Port=2  PortName=DisplayLink
  wires:
  Bus Element In1/1 -> Rideshare PCB/1(RideshareRail_3v3)

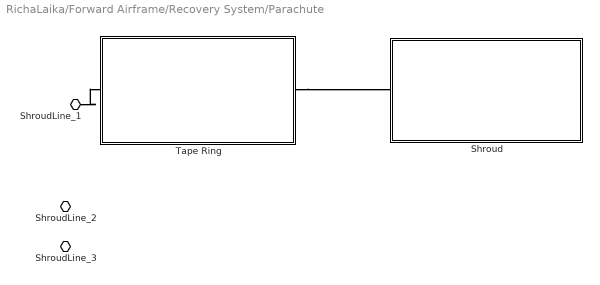
== system RichaLaika/Forward Airframe/Recovery System/Parachute ==
  Shroud : Subsystem
      settings: PortSchema="{\"entries\":[{\"content\":{\"headerSize\":26,\"margin\":15,\"minimumSpacing\":25,\"sides\":[{\"content\":{\"connectorIds\":[\"LConn1\"]},\"type\":\"ConnectorPlacement.EquallySpacedRectSide\",\"uuid\":\"03e957df-4bae-46ab-9d0d-48f80a496ac5\"},{\"content\":{\"side\":\"RIGHT\"},\"type\":\"ConnectorPlacement.EquallySpacedRectSide\",\"uuid\":\"d2433d43-ba0e-4345-8a8e-99b57dcef125\"},{\"content\":{\"side\":\"TOP\"},\"type\":\"ConnectorPlacement.EquallySpacedRectSide\",\"uuid\":\"84844adf-0e3d-439c-a28c-7cf27e8d243a\"}]},\"type\":\"ConnectorPlacement.EquallySpacedConnector\",\"uuid\":\"9b26577b-50b2-4983-8f3c-4df87f23ba49\"}],\"packageUris\":[\"http://schema.mathworks.com/mf0/Connector/R2020b\"],\"version\":\"1.0\"}"
  Tape Ring : Subsystem
      settings: PortSchema="{\"entries\":[{\"content\":{\"headerSize\":26,\"margin\":15,\"minimumSpacing\":25,\"sides\":[{\"content\":{\"connectorIds\":[\"LConn1\"]},\"type\":\"ConnectorPlacement.EquallySpacedRectSide\",\"uuid\":\"03e957df-4bae-46ab-9d0d-48f80a496ac5\"},{\"content\":{\"connectorIds\":[\"RConn1\"],\"side\":\"RIGHT\"},\"type\":\"ConnectorPlacement.EquallySpacedRectSide\",\"uuid\":\"d2433d43-ba0e-4345-8a8e-99b57dcef125\"},{\"content\":{\"side\":\"TOP\"},\"type\":\"ConnectorPlacement.EquallySpacedRectSide\",\"uuid\":\"84844adf-0e3d-439c-a28c-7cf27e8d243a\"}]},\"type\":\"ConnectorPlacement.EquallySpacedConnector\",\"uuid\":\"9b26577b-50b2-4983-8f3c-4df87f23ba49\"}],\"packageUris\":[\"http://schema.mathworks.com/mf0/Connector/R2020b\"],\"version\":\"1.0\"}"
  ShroudLine_1 : PMIOPort  Side=Left
  ShroudLine_2 : PMIOPort  Port=2  Side=Left
  ShroudLine_3 : PMIOPort  Port=3  Side=Left
  connections:
  ShroudLine_1/RConn1 -- Tape Ring/LConn1
  Tape Ring/RConn1 -- Shroud/LConn1

== system RichaLaika/Forward Airframe/Recovery System/Recovery Hardware ==

== system RichaLaika/Forward Airframe/Recovery System/Shock Chord ==
  ShockCrd : PMIOPort  Side=Left

== system RichaLaika/Forward Airframe/Payload Module/Customer Payload Bay/Customer Payload ==
  In Bus Element1 : Inport  PortName=Customer Payload Connector

== system RichaLaika/Forward Airframe/Payload Module/Customer Payload Bay/Male XT30 Connector ==
  Bus Element In1 : Inport  PortName=CustomerBus_3v7
  Bus Element Out1 : Outport  PortName=Customer Payload Connector

== system RichaLaika/Forward Airframe/Payload Module/Power Subsystem/Custom PCB ==
  Bus Element In1 : Inport  PortName=InBus

== system RichaLaika/Forward Airframe/Payload Module/Power Subsystem/MainBattery_3p74_4500mAh ==
  Bus Element Out1 : Outport  PortName=OutBus

== system RichaLaika/Forward Airframe/Payload Module/Power Subsystem/Regulator_Customer ==
  Bus Element In2 : Inport  PortName=InBus
  Bus Element Out1 : Outport  PortName=Regulator_3v7_Customer.Out

== system RichaLaika/Forward Airframe/Payload Module/Power Subsystem/Regulator_Rideshare ==
  Bus Element In2 : Inport  PortName=InBus
  Bus Element Out1 : Outport  PortName=Regulator_3v3_Rideshare.Out

== system RichaLaika/Forward Airframe/Payload Module/Power Subsystem/Screw Switch ==
  Bus Element In1 : Inport  PortName=InBus
  Bus Element Out1 : Outport  PortName=OutBus

== system RichaLaika/Forward Airframe/Payload Module/Rideshare Payload Bay/Ride Share Payload ==
  Altitude Detection System : Subsystem
      settings: PortSchema="{\"entries\":[{\"content\":{\"headerSize\":26,\"margin\":15,\"minimumSpacing\":25,\"sides\":[{\"content\":{},\"type\":\"ConnectorPlacement.EquallySpacedRectSide\",\"uuid\":\"6f4db608-f49c-4d1a-85cc-b66ec62c2f96\"},{\"content\":{\"side\":\"RIGHT\"},\"type\":\"ConnectorPlacement.EquallySpacedRectSide\",\"uuid\":\"3e275c67-1c5c-46cd-973f-75adcfca9e5d\"},{\"content\":{\"side\":\"TOP\"},\"type\":\"ConnectorPlacement.EquallySpacedRectSide\",\"uuid\":\"88fdcd36-c2bf-423f-a1bd-8e2b1c2ac438\"}]},\"type\":\"ConnectorPlacement.EquallySpacedConnector\",\"uuid\":\"596a3d77-8add-49e5-be48-e23e6a2b115a\"}],\"packageUris\":[\"http://schema.mathworks.com/mf0/Connector/R2020b\"],\"version\":\"1.0\"}"
  Chosen Data Collection : Subsystem
      settings: PortSchema="{\"entries\":[{\"content\":{\"headerSize\":26,\"margin\":15,\"minimumSpacing\":25,\"sides\":[{\"content\":{},\"type\":\"ConnectorPlacement.EquallySpacedRectSide\",\"uuid\":\"6f4db608-f49c-4d1a-85cc-b66ec62c2f96\"},{\"content\":{\"side\":\"RIGHT\"},\"type\":\"ConnectorPlacement.EquallySpacedRectSide\",\"uuid\":\"3e275c67-1c5c-46cd-973f-75adcfca9e5d\"},{\"content\":{\"side\":\"TOP\"},\"type\":\"ConnectorPlacement.EquallySpacedRectSide\",\"uuid\":\"88fdcd36-c2bf-423f-a1bd-8e2b1c2ac438\"}]},\"type\":\"ConnectorPlacement.EquallySpacedConnector\",\"uuid\":\"596a3d77-8add-49e5-be48-e23e6a2b115a\"}],\"packageUris\":[\"http://schema.mathworks.com/mf0/Connector/R2020b\"],\"version\":\"1.0\"}"
  Printed Circuit Board : Subsystem
      settings: PortSchema="{\"entries\":[{\"content\":{\"headerSize\":26,\"margin\":15,\"minimumSpacing\":25,\"sides\":[{\"content\":{},\"type\":\"ConnectorPlacement.EquallySpacedRectSide\",\"uuid\":\"6f4db608-f49c-4d1a-85cc-b66ec62c2f96\"},{\"content\":{\"side\":\"RIGHT\"},\"type\":\"ConnectorPlacement.EquallySpacedRectSide\",\"uuid\":\"3e275c67-1c5c-46cd-973f-75adcfca9e5d\"},{\"content\":{\"side\":\"TOP\"},\"type\":\"ConnectorPlacement.EquallySpacedRectSide\",\"uuid\":\"88fdcd36-c2bf-423f-a1bd-8e2b1c2ac438\"}]},\"type\":\"ConnectorPlacement.EquallySpacedConnector\",\"uuid\":\"596a3d77-8add-49e5-be48-e23e6a2b115a\"}],\"packageUris\":[\"http://schema.mathworks.com/mf0/Connector/R2020b\"],\"version\":\"1.0\"}"

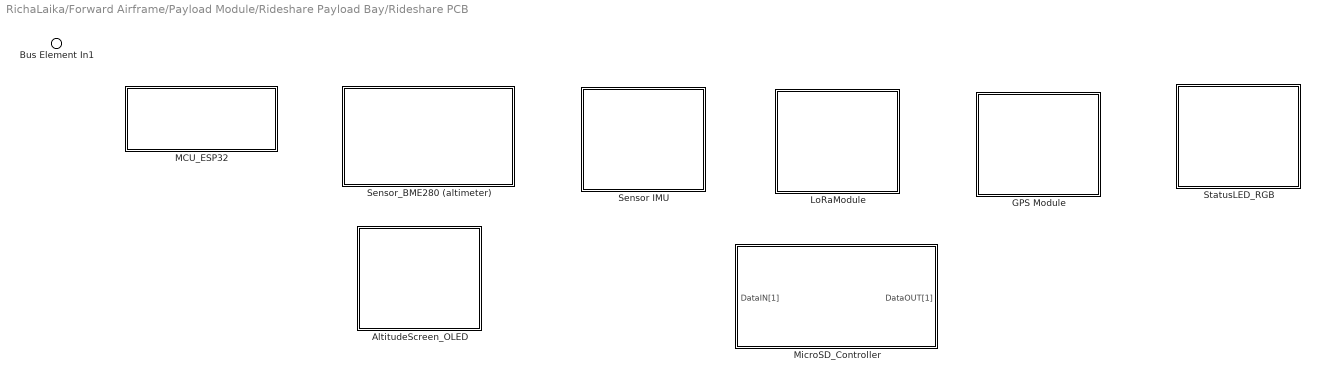
== system RichaLaika/Forward Airframe/Payload Module/Rideshare Payload Bay/Rideshare PCB ==
  Bus Element In1 : Inport  PortName=RideshareRail_3v3
  AltitudeScreen_OLED : Subsystem
      settings: PortSchema="{\"entries\":[{\"content\":{\"headerSize\":26,\"margin\":15,\"minimumSpacing\":25,\"sides\":[{\"content\":{},\"type\":\"ConnectorPlacement.EquallySpacedRectSide\",\"uuid\":\"b8130898-a228-4777-928b-c45fd71fae12\"},{\"content\":{\"side\":\"RIGHT\"},\"type\":\"ConnectorPlacement.EquallySpacedRectSide\",\"uuid\":\"2e534d82-eb77-4958-a6c7-3df50b0f76b8\"},{\"content\":{\"side\":\"TOP\"},\"type\":\"ConnectorPlacement.EquallySpacedRectSide\",\"uuid\":\"3377e7dd-a415-4e95-88ef-4d0f5ef1cb04\"}]},\"type\":\"ConnectorPlacement.EquallySpacedConnector\",\"uuid\":\"f74309f9-da3e-4b22-b86a-0a2c471e6b03\"}],\"packageUris\":[\"http://schema.mathworks.com/mf0/Connector/R2020b\"],\"version\":\"1.0\"}"
  GPS Module : Subsystem
      settings: PortSchema="{\"entries\":[{\"content\":{\"headerSize\":26,\"margin\":15,\"minimumSpacing\":25,\"sides\":[{\"content\":{},\"type\":\"ConnectorPlacement.EquallySpacedRectSide\",\"uuid\":\"b8130898-a228-4777-928b-c45fd71fae12\"},{\"content\":{\"side\":\"RIGHT\"},\"type\":\"ConnectorPlacement.EquallySpacedRectSide\",\"uuid\":\"2e534d82-eb77-4958-a6c7-3df50b0f76b8\"},{\"content\":{\"side\":\"TOP\"},\"type\":\"ConnectorPlacement.EquallySpacedRectSide\",\"uuid\":\"3377e7dd-a415-4e95-88ef-4d0f5ef1cb04\"}]},\"type\":\"ConnectorPlacement.EquallySpacedConnector\",\"uuid\":\"f74309f9-da3e-4b22-b86a-0a2c471e6b03\"}],\"packageUris\":[\"http://schema.mathworks.com/mf0/Connector/R2020b\"],\"version\":\"1.0\"}"
  LoRaModule : Subsystem
      settings: PortSchema="{\"entries\":[{\"content\":{\"headerSize\":26,\"margin\":15,\"minimumSpacing\":25,\"sides\":[{\"content\":{},\"type\":\"ConnectorPlacement.EquallySpacedRectSide\",\"uuid\":\"b8130898-a228-4777-928b-c45fd71fae12\"},{\"content\":{\"side\":\"RIGHT\"},\"type\":\"ConnectorPlacement.EquallySpacedRectSide\",\"uuid\":\"2e534d82-eb77-4958-a6c7-3df50b0f76b8\"},{\"content\":{\"side\":\"TOP\"},\"type\":\"ConnectorPlacement.EquallySpacedRectSide\",\"uuid\":\"3377e7dd-a415-4e95-88ef-4d0f5ef1cb04\"}]},\"type\":\"ConnectorPlacement.EquallySpacedConnector\",\"uuid\":\"f74309f9-da3e-4b22-b86a-0a2c471e6b03\"}],\"packageUris\":[\"http://schema.mathworks.com/mf0/Connector/R2020b\"],\"version\":\"1.0\"}"
  MCU_ESP32 : Subsystem
      settings: PortSchema="{\"entries\":[{\"content\":{\"headerSize\":26,\"margin\":15,\"minimumSpacing\":25,\"sides\":[{\"content\":{},\"type\":\"ConnectorPlacement.EquallySpacedRectSide\",\"uuid\":\"31a1afce-5e8d-4ecd-8541-15d1c40c1f45\"},{\"content\":{\"side\":\"RIGHT\"},\"type\":\"ConnectorPlacement.EquallySpacedRectSide\",\"uuid\":\"3ed7ed21-4334-432f-9367-bfee11c65601\"},{\"content\":{\"side\":\"TOP\"},\"type\":\"ConnectorPlacement.EquallySpacedRectSide\",\"uuid\":\"099656eb-739b-474e-8ddd-dbd0ceba9a2b\"}]},\"type\":\"ConnectorPlacement.EquallySpacedConnector\",\"uuid\":\"a8320310-5044-4b61-8848-b99dff184188\"}],\"packageUris\":[\"http://schema.mathworks.com/mf0/Connector/R2020b\"],\"version\":\"1.0\"}"
  MicroSD_Controller : Subsystem
      settings: PortSchema="{\"entries\":[{\"content\":{\"headerSize\":26,\"margin\":15,\"minimumSpacing\":25,\"sides\":[{\"content\":{\"connectorIds\":[\"In1\"]},\"type\":\"ConnectorPlacement.EquallySpacedRectSide\",\"uuid\":\"6f4db608-f49c-4d1a-85cc-b66ec62c2f96\"},{\"content\":{\"connectorIds\":[\"Out1\"],\"side\":\"RIGHT\"},\"type\":\"ConnectorPlacement.EquallySpacedRectSide\",\"uuid\":\"3e275c67-1c5c-46cd-973f-75adcfca9e5d\"},{\"content\":{\"side\":\"TOP\"},\"type\":\"ConnectorPlacement.EquallySpacedRectSide\",\"uuid\":\"88fdcd36-c2bf-423f-a1bd-8e2b1c2ac438\"}]},\"type\":\"ConnectorPlacement.EquallySpacedConnector\",\"uuid\":\"596a3d77-8add-49e5-be48-e23e6a2b115a\"}],\"packageUris\":[\"http://schema.mathworks.com/mf0/Connector/R2020b\"],\"version\":\"1.0\"}"
  Sensor IMU : Subsystem
      settings: PortSchema="{\"entries\":[{\"content\":{\"headerSize\":26,\"margin\":15,\"minimumSpacing\":25,\"sides\":[{\"content\":{},\"type\":\"ConnectorPlacement.EquallySpacedRectSide\",\"uuid\":\"b8130898-a228-4777-928b-c45fd71fae12\"},{\"content\":{\"side\":\"RIGHT\"},\"type\":\"ConnectorPlacement.EquallySpacedRectSide\",\"uuid\":\"2e534d82-eb77-4958-a6c7-3df50b0f76b8\"},{\"content\":{\"side\":\"TOP\"},\"type\":\"ConnectorPlacement.EquallySpacedRectSide\",\"uuid\":\"3377e7dd-a415-4e95-88ef-4d0f5ef1cb04\"}]},\"type\":\"ConnectorPlacement.EquallySpacedConnector\",\"uuid\":\"f74309f9-da3e-4b22-b86a-0a2c471e6b03\"}],\"packageUris\":[\"http://schema.mathworks.com/mf0/Connector/R2020b\"],\"version\":\"1.0\"}"
  Sensor_BME280 (altimeter) : Subsystem
      settings: PortSchema="{\"entries\":[{\"content\":{\"headerSize\":26,\"margin\":15,\"minimumSpacing\":25,\"sides\":[{\"content\":{},\"type\":\"ConnectorPlacement.EquallySpacedRectSide\",\"uuid\":\"b8130898-a228-4777-928b-c45fd71fae12\"},{\"content\":{\"side\":\"RIGHT\"},\"type\":\"ConnectorPlacement.EquallySpacedRectSide\",\"uuid\":\"2e534d82-eb77-4958-a6c7-3df50b0f76b8\"},{\"content\":{\"side\":\"TOP\"},\"type\":\"ConnectorPlacement.EquallySpacedRectSide\",\"uuid\":\"3377e7dd-a415-4e95-88ef-4d0f5ef1cb04\"}]},\"type\":\"ConnectorPlacement.EquallySpacedConnector\",\"uuid\":\"f74309f9-da3e-4b22-b86a-0a2c471e6b03\"}],\"packageUris\":[\"http://schema.mathworks.com/mf0/Connector/R2020b\"],\"version\":\"1.0\"}"
  StatusLED_RGB : Subsystem
      settings: PortSchema="{\"entries\":[{\"content\":{\"headerSize\":26,\"margin\":15,\"minimumSpacing\":25,\"sides\":[{\"content\":{},\"type\":\"ConnectorPlacement.EquallySpacedRectSide\",\"uuid\":\"b8130898-a228-4777-928b-c45fd71fae12\"},{\"content\":{\"side\":\"RIGHT\"},\"type\":\"ConnectorPlacement.EquallySpacedRectSide\",\"uuid\":\"2e534d82-eb77-4958-a6c7-3df50b0f76b8\"},{\"content\":{\"side\":\"TOP\"},\"type\":\"ConnectorPlacement.EquallySpacedRectSide\",\"uuid\":\"3377e7dd-a415-4e95-88ef-4d0f5ef1cb04\"}]},\"type\":\"ConnectorPlacement.EquallySpacedConnector\",\"uuid\":\"f74309f9-da3e-4b22-b86a-0a2c471e6b03\"}],\"packageUris\":[\"http://schema.mathworks.com/mf0/Connector/R2020b\"],\"version\":\"1.0\"}"

== system RichaLaika/Forward Airframe/Recovery System/Parachute/Shroud ==
  ShroudLines[2] : PMIOPort  Side=Left

== system RichaLaika/Forward Airframe/Recovery System/Parachute/Tape Ring ==
  ShroudLines_1 : PMIOPort  Side=Left
  ShroudLines[2] : PMIOPort  Port=2  Side=Right

== system RichaLaika/Forward Airframe/Payload Module/Rideshare Payload Bay/Ride Share Payload/Altitude Detection System ==

== system RichaLaika/Forward Airframe/Payload Module/Rideshare Payload Bay/Ride Share Payload/Chosen Data Collection ==

== system RichaLaika/Forward Airframe/Payload Module/Rideshare Payload Bay/Ride Share Payload/Printed Circuit Board ==

== system RichaLaika/Forward Airframe/Payload Module/Rideshare Payload Bay/Rideshare PCB/AltitudeScreen_OLED ==

== system RichaLaika/Forward Airframe/Payload Module/Rideshare Payload Bay/Rideshare PCB/GPS Module ==

== system RichaLaika/Forward Airframe/Payload Module/Rideshare Payload Bay/Rideshare PCB/LoRaModule ==

== system RichaLaika/Forward Airframe/Payload Module/Rideshare Payload Bay/Rideshare PCB/MCU_ESP32 ==

== system RichaLaika/Forward Airframe/Payload Module/Rideshare Payload Bay/Rideshare PCB/MicroSD_Controller ==
  Bus Element In1 : Inport  PortName=DataIN[1]
  Bus Element Out1 : Outport  PortName=DataOUT[1]

== system RichaLaika/Forward Airframe/Payload Module/Rideshare Payload Bay/Rideshare PCB/Sensor IMU ==

== system RichaLaika/Forward Airframe/Payload Module/Rideshare Payload Bay/Rideshare PCB/Sensor_BME280 (altimeter) ==

== system RichaLaika/Forward Airframe/Payload Module/Rideshare Payload Bay/Rideshare PCB/StatusLED_RGB ==
